simulink model "sampleModel1429"  (R2023a)
settings: Solver=VariableStepAuto  StartTime=0.0  StopTime=10.0  RelTol=1e-3
libraries: hdlsllib x6, simulink x1
settings Model: Creator=user1  LastModifiedBy=user1

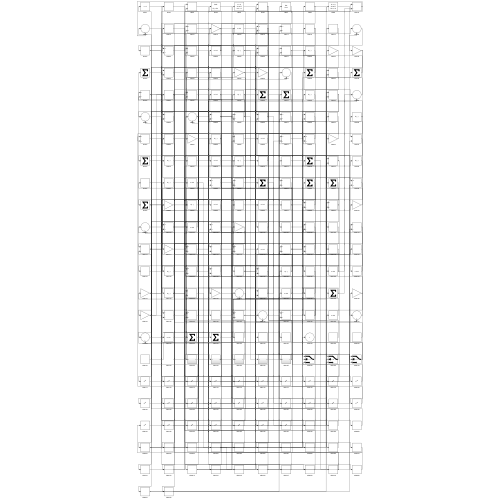
[thumbnail: Simulink's stored preview of the top-level diagram]
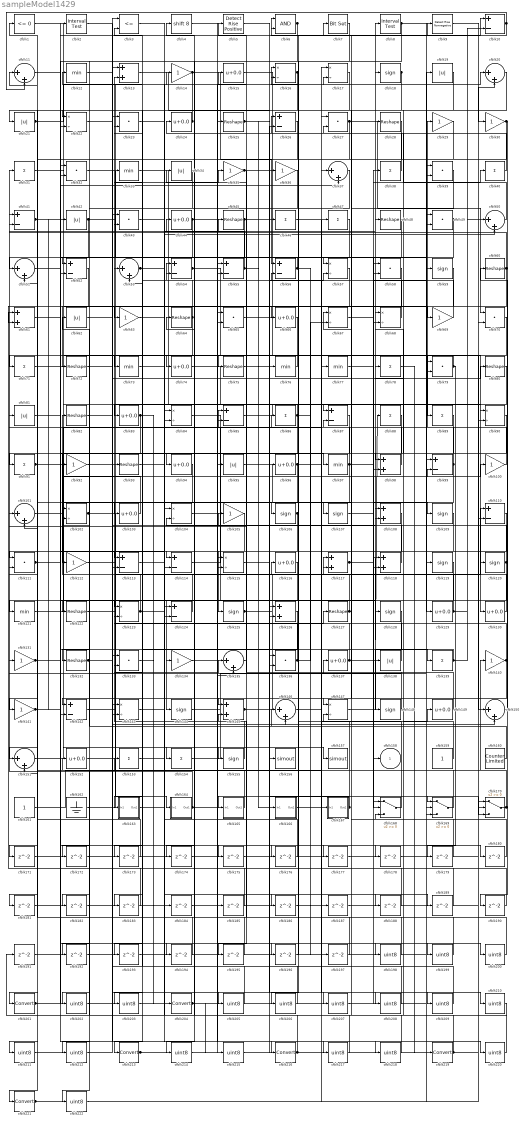
== system sampleModel1429 ==
  cfblk1 : hdlsllib/Logic and Bit Operations/Compare To Zero  relop=<=  OutDataTypeStr=boolean
  cfblk{10,26,41,52,54..56,85,87,99,110,113..114,124,142} (15 alike) : Sum  Inputs=+-
  cfblk{14,29..30,35..36,63,69,92,100,105,112,131,134,140..141} (15 alike) : Gain
  cfblk{11,20,37,50..51,53,101,135,146,150..151} (11 alike) : Sum  Inputs=|++
  cfblk{16..17,22,57,67..68,84,90,102,104,115,123,143,147} (14 alike) : Product  Inputs=*/  RndMeth=Zero  SaturateOnIntegerOverflow=on
  cfblk{15,24,44,66,74,83,94,96,103,116,129..130,137,149,152} (15 alike) : Bias  Bias=0.0  SaturateOnIntegerOverflow=off
  cfblk{18,59,106..107,109,119..120,125,128,144,148,155} (12 alike) : Signum
  cfblk{13,61,98,108,117..118,126,145} (8 alike) : Sum
  cfblk{23,27,32,39,43,49,58,65,70,79,111,133,136} (13 alike) : DotProduct  OutDataTypeStr=Inherit: Inherit via internal rule
  cfblk{12,33,73,76..77,97,121} (7 alike) : MinMax
  cfblk{25,28,45,48,60,64,72,75,80,82,93,122,127,132} (14 alike) : Reshape
  cfblk{19,21,34,42,62,81,95,138} (8 alike) : Abs  SaturateOnIntegerOverflow=off
  cfblk{31,38,40,46..47,71,78,86,88..89,91,139,153..154} (14 alike) : Sum  Inputs=+
  cfblk156 : ToWorkspace  VariableName=simout  SaveFormat=Timeseries  SampleTime=-1
  cfblk157 : ToWorkspace  VariableName=simout  SaveFormat=Timeseries  SampleTime=-1
  cfblk159 : Constant  SampleTime=-1
  cfblk160 : hdlsllib/Sources/Counter Limited  uplimit=7  tsamp=-1
  cfblk161 : Constant  SampleTime=-1
  cfblk162 : Ground
  cfblk163 : Subsystem
      settings: LibrarySourceBlock=|
      | hdlsllib/Ports &
      | Subsystems/Subsystem
  cfblk164 : Subsystem
      settings: LibrarySourceBlock=|
      | hdlsllib/Ports &
      | Subsystems/Subsystem
  cfblk165 : Subsystem
      settings: LibrarySourceBlock=|
      | hdlsllib/Ports &
      | Subsystems/Subsystem
  cfblk166 : Subsystem
      settings: LibrarySourceBlock=|
      | hdlsllib/Ports &
      | Subsystems/Subsystem
  cfblk167 : Subsystem
      settings: LibrarySourceBlock=|
      | hdlsllib/Ports &
      | Subsystems/Subsystem
  cfblk168 : Switch  SaturateOnIntegerOverflow=off  InputSameDT=off
  cfblk169 : Switch  SaturateOnIntegerOverflow=off  InputSameDT=off
  cfblk170 : Switch  SaturateOnIntegerOverflow=off  InputSameDT=off
  cfblk{171..197} (27 alike) : Delay  SampleTime=1
  cfblk{198..200,202..203,205..212,214..215,217..218,220,222} (19 alike) : DataTypeConversion  OutDataTypeStr=uint8  SaturateOnIntegerOverflow=off  RndMeth=Floor
  cfblk2 : hdlsllib/Logic and Bit Operations/Interval Test  IntervalClosedRight=on  uplimit=0.5  IntervalClosedLeft=on  lowlimit=-0.5  OutDataTypeStr=boolean
  cfblk{201,204,213,216,219,221} (6 alike) : DataTypeConversion  SaturateOnIntegerOverflow=off  RndMeth=Floor
  cfblk3 : RelationalOperator  Operator=<=  OutDataTypeStr=boolean  InputSameDT=off
  cfblk4 : ArithShift  BitShiftNumber=8
  cfblk5 : hdlsllib/Logic and Bit Operations/Detect Rise Positive  vinit=0  OutDataTypeStr=boolean
  cfblk6 : Logic  AllPortsSameDT=off  OutDataTypeStr=boolean
  cfblk7 : simulink/Logic and Bit Operations/Bit Set  iBit=0
      settings: LibrarySourceBlock=|
      | hdlsllib/Logic and Bit
      | Operations/Bit Set
  cfblk8 : hdlsllib/Logic and Bit Operations/Interval Test  IntervalClosedRight=on  uplimit=0.5  IntervalClosedLeft=on  lowlimit=-0.5  OutDataTypeStr=boolean
  cfblk9 : hdlsllib/Logic and Bit Operations/Detect Rise Nonnegative  vinit=0  OutDataTypeStr=boolean
  cfblk158 : Outport  VectorParamsAs1DForOutWhenUnconnected=off
  wires:
  cfblk154/1 -> cfblk137/1
  cfblk122/1 -> cfblk85/1
  cfblk165/1(Out1) -> cfblk11/1
  cfblk164/1(Out1) -> cfblk31/1, cfblk135/2
  cfblk136/1 -> cfblk13/2, cfblk67/2
  cfblk83/1 -> cfblk151/2, cfblk184/1
  cfblk16/1 -> cfblk124/2, cfblk193/1
  cfblk112/1 -> cfblk35/1
  cfblk25/1 -> cfblk76/1, cfblk170/3
  cfblk65/1 -> cfblk130/1
  cfblk108/1 -> cfblk125/1
  cfblk71/1 -> cfblk106/1
  cfblk40/1 -> cfblk7/1
  cfblk74/1 -> cfblk156/1
  cfblk124/1 -> cfblk82/1
  cfblk84/1 -> cfblk167/1(In1)
  cfblk147/1 -> cfblk8/1
  cfblk161/1 -> cfblk77/1
  cfblk91/1 -> cfblk155/1, cfblk114/2
  cfblk102/1 -> cfblk164/1(In1), cfblk79/2
  cfblk33/1 -> cfblk85/2
  cfblk170/1 -> cfblk140/1, cfblk153/1
  cfblk110/1 -> cfblk111/1
  cfblk109/1 -> cfblk121/1
  cfblk155/1 -> cfblk53/1
  cfblk120/1 -> cfblk44/1, cfblk214/1
  cfblk81/1 -> cfblk97/1
  cfblk8/1 -> cfblk119/1, cfblk206/1
  cfblk18/1 -> cfblk147/1, cfblk51/2
  cfblk42/1 -> cfblk20/1, cfblk146/2, cfblk52/1
  cfblk32/1 -> cfblk129/1
  cfblk1/1 -> cfblk90/1
  cfblk79/1 -> cfblk74/1, cfblk179/1
  cfblk137/1 -> cfblk88/1, cfblk86/1
  cfblk66/1 -> cfblk71/1
  cfblk162/1 -> cfblk127/1
  cfblk60/1 -> cfblk114/1, cfblk41/2
  cfblk98/1 -> cfblk54/1
  cfblk52/1 -> cfblk72/1
  cfblk47/1 -> cfblk221/1
  cfblk39/1 -> cfblk107/1
  cfblk86/1 -> cfblk83/1, cfblk113/2, cfblk187/1
  cfblk128/1 -> cfblk148/1
  cfblk92/1 -> cfblk94/1
  cfblk116/1 -> cfblk144/1
  cfblk64/1 -> cfblk33/1, cfblk142/2
  cfblk87/1 -> cfblk91/1
  cfblk113/1 -> cfblk48/1
  cfblk58/1 -> cfblk201/1
  cfblk15/1 -> cfblk150/1
  cfblk27/1 -> cfblk70/1, cfblk211/1
  cfblk6/1 -> cfblk134/1, cfblk22/2
  cfblk72/1 -> cfblk93/1
  cfblk29/1 -> cfblk73/1
  cfblk126/1 -> cfblk213/1
  cfblk67/1 -> cfblk38/1
  cfblk93/1 -> cfblk45/1
  cfblk75/1 -> cfblk150/2
  cfblk100/1 -> cfblk64/1
  cfblk9/1 -> cfblk30/1
  cfblk169/1 -> cfblk117/1
  cfblk127/1 -> cfblk116/1, cfblk67/1
  cfblk68/1 -> cfblk12/1
  cfblk30/1 -> cfblk190/1, cfblk212/1
  cfblk14/1 -> cfblk56/1, cfblk102/1
  cfblk78/1 -> cfblk219/1
  cfblk41/1 -> cfblk168/1, cfblk194/1
  cfblk22/1 -> cfblk9/1
  cfblk146/1 -> cfblk170/2
  cfblk11/1 -> cfblk57/1
  cfblk160/1 -> cfblk62/1
  cfblk82/1 -> cfblk154/1
  cfblk44/1 -> cfblk151/1, cfblk200/1
  cfblk148/1 -> cfblk135/1, cfblk34/1, cfblk123/2
  cfblk168/1 -> cfblk81/1
  cfblk145/1 -> cfblk110/1, cfblk57/2
  cfblk115/1 -> cfblk99/2
  cfblk99/1 -> cfblk29/1, cfblk168/2
  cfblk53/1 -> cfblk50/2, cfblk173/1
  cfblk166/1(Out1) -> cfblk149/1
  cfblk50/1 -> cfblk28/1
  cfblk142/1 -> cfblk120/1
  cfblk12/1 -> cfblk69/1
  cfblk73/1 -> cfblk18/1
  cfblk20/1 -> cfblk132/1
  cfblk76/1 -> cfblk75/1
  cfblk97/1 -> cfblk141/1, cfblk109/1, cfblk16/2
  cfblk77/1 -> cfblk59/1
  cfblk114/1 -> cfblk17/1
  cfblk130/1 -> cfblk3/2
  cfblk159/1 -> cfblk108/1
  cfblk95/1 -> cfblk118/1
  cfblk24/1 -> cfblk21/1, cfblk22/1
  cfblk121/1 -> cfblk36/1
  cfblk131/1 -> cfblk2/1, cfblk10/1
  cfblk118/1 -> cfblk4/1
  cfblk163/1(Out1) -> cfblk105/1
  cfblk138/1 -> cfblk15/1
  cfblk31/1 -> cfblk84/2
  cfblk59/1 -> cfblk66/1
  cfblk96/1 -> cfblk142/1, cfblk209/1
  cfblk37/1 -> cfblk115/1
  cfblk55/1 -> cfblk5/1, cfblk41/1, cfblk166/1(In1)
  cfblk140/1 -> cfblk26/1, cfblk182/1
  cfblk106/1 -> cfblk16/1, cfblk202/1
  cfblk129/1 -> cfblk123/1, cfblk68/1, cfblk10/2
  cfblk151/1 -> cfblk157/1
  cfblk123/1 -> cfblk80/1, cfblk102/2
  cfblk104/1 -> cfblk216/1
  cfblk38/1 -> cfblk24/1
  cfblk54/1 -> cfblk89/1, cfblk136/2, cfblk17/2
  cfblk10/1 -> cfblk11/2, cfblk6/2
  cfblk45/1 -> cfblk103/1, cfblk68/2
  cfblk69/1 -> cfblk6/1
  cfblk167/1(Out1) -> cfblk131/1, cfblk165/1(In1)
  cfblk13/1 -> cfblk96/1
  cfblk139/1 -> cfblk138/1, cfblk50/1
  cfblk125/1 -> cfblk79/1, cfblk180/1
  cfblk49/1 -> cfblk118/2, cfblk63/1
  cfblk132/1 -> cfblk108/2, cfblk178/1
  cfblk90/1 -> cfblk112/1
  cfblk48/1 -> cfblk163/1(In1)
  cfblk144/1 -> cfblk19/1
  cfblk85/1 -> cfblk87/1
  cfblk103/1 -> cfblk92/1
  cfblk57/1 -> cfblk61/2
  cfblk133/1 -> cfblk204/1
  cfblk17/1 -> cfblk55/2
  cfblk19/1 -> cfblk98/1
  cfblk7/1 -> cfblk122/1
  cfblk149/1 -> cfblk101/1
  cfblk35/1 -> cfblk145/1, cfblk169/1
  cfblk141/1 -> cfblk42/1, cfblk177/1
  cfblk21/1 -> cfblk14/1, cfblk128/1
  cfblk101/1 -> cfblk26/2
  cfblk111/1 -> cfblk37/2, cfblk139/1
  cfblk150/1 -> cfblk60/1
  cfblk107/1 -> cfblk40/1
  cfblk117/1 -> cfblk98/2, cfblk100/1
  cfblk34/1 -> cfblk113/1
  cfblk94/1 -> cfblk101/2
  cfblk28/1 -> cfblk32/2
  cfblk152/1 -> cfblk25/1
  cfblk56/1 -> cfblk51/1, cfblk197/1
  cfblk119/1 -> cfblk171/1
  cfblk171/1 -> cfblk90/2
  cfblk89/1 -> cfblk172/1
  cfblk172/1 -> cfblk37/1
  cfblk173/1 -> cfblk111/2
  cfblk80/1 -> cfblk174/1
  cfblk174/1 -> cfblk136/1
  cfblk2/1 -> cfblk175/1
  cfblk3/1 -> cfblk176/1
  cfblk176/1 -> cfblk84/1
  cfblk177/1 -> cfblk117/2
  cfblk178/1 -> cfblk110/2
  cfblk179/1 -> cfblk87/2
  cfblk180/1 -> cfblk168/3
  cfblk26/1 -> cfblk181/1
  cfblk181/1 -> cfblk55/1
  cfblk182/1 -> cfblk115/2
  cfblk88/1 -> cfblk183/1
  cfblk183/1 -> cfblk61/1
  cfblk184/1 -> cfblk170/1
  cfblk4/1 -> cfblk185/1
  cfblk185/1 -> cfblk53/2
  cfblk63/1 -> cfblk186/1
  cfblk186/1 -> cfblk146/1
  cfblk187/1 -> cfblk169/2
  cfblk46/1 -> cfblk188/1
  cfblk188/1 -> cfblk147/2
  cfblk134/1 -> cfblk189/1
  cfblk189/1 -> cfblk13/1
  cfblk190/1 -> cfblk54/2
  cfblk191/1 -> cfblk39/2
  cfblk36/1 -> cfblk192/1
  cfblk193/1 -> cfblk99/1
  cfblk194/1 -> cfblk1/1
  cfblk135/1 -> cfblk195/1
  cfblk195/1 -> cfblk32/1
  cfblk51/1 -> cfblk196/1
  cfblk196/1 -> cfblk56/2
  cfblk197/1 -> cfblk145/2
  cfblk43/1 -> cfblk198/1
  cfblk198/1 -> cfblk65/1
  cfblk5/1 -> cfblk199/1
  cfblk199/1 -> cfblk43/1
  cfblk200/1 -> cfblk43/2
  cfblk201/1 -> cfblk52/2, cfblk46/1, cfblk3/1
  cfblk202/1 -> cfblk58/1
  cfblk70/1 -> cfblk203/1
  cfblk203/1 -> cfblk58/2
  cfblk204/1 -> cfblk169/3, cfblk158/1, cfblk215/1
  cfblk62/1 -> cfblk205/1
  cfblk205/1 -> cfblk133/1
  cfblk206/1 -> cfblk133/2
  cfblk23/1 -> cfblk207/1
  cfblk207/1 -> cfblk39/1
  cfblk175/1 -> cfblk208/1
  cfblk208/1 -> cfblk23/1
  cfblk209/1 -> cfblk23/2
  cfblk143/1 -> cfblk210/1
  cfblk210/1 -> cfblk191/1
  cfblk211/1 -> cfblk143/1
  cfblk212/1 -> cfblk143/2
  cfblk213/1 -> cfblk65/2, cfblk95/1, cfblk27/1
  cfblk214/1 -> cfblk126/1
  cfblk215/1 -> cfblk126/2
  cfblk216/1 -> cfblk70/2, cfblk49/1, cfblk152/1
  cfblk61/1 -> cfblk217/1
  cfblk217/1 -> cfblk104/1
  cfblk192/1 -> cfblk218/1
  cfblk218/1 -> cfblk104/2
  cfblk219/1 -> cfblk27/2, cfblk124/1
  cfblk153/1 -> cfblk220/1
  cfblk220/1 -> cfblk78/1
  cfblk221/1 -> cfblk49/2, cfblk20/2
  cfblk105/1 -> cfblk222/1
  cfblk222/1 -> cfblk47/1

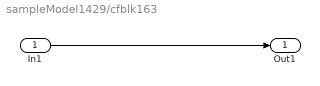
== system sampleModel1429/cfblk163 ==
  In1 : Inport
  Out1 : Outport
  wires:
  In1/1 -> Out1/1

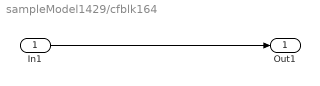
== system sampleModel1429/cfblk164 ==
  In1 : Inport
  Out1 : Outport
  wires:
  In1/1 -> Out1/1

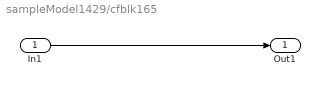
== system sampleModel1429/cfblk165 ==
  In1 : Inport
  Out1 : Outport
  wires:
  In1/1 -> Out1/1

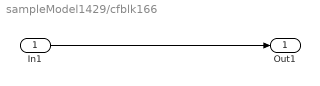
== system sampleModel1429/cfblk166 ==
  In1 : Inport
  Out1 : Outport
  wires:
  In1/1 -> Out1/1

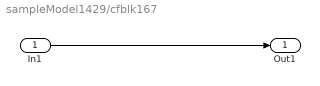
== system sampleModel1429/cfblk167 ==
  In1 : Inport
  Out1 : Outport
  wires:
  In1/1 -> Out1/1
